simulink model "lin_kw_sim"  (R2021a)
settings: Solver=ode5  StartTime=0.0  StopTime=T  FixedStep=sim_step  RelTol=1e-3  AbsTol=1e-6
values from neighbouring files (symbols this model uses):
  f = Fk/(M*g)    [ideal_pendulum.m]    (also in lin_kw.m = 0.00027344; rms_calc.m = 1e-05)
  g = 9.81    [ideal_pendulum.m]    (also in lin_kw.m; non_lin_inv_pend_sim_real.m; non_lin_inverted_pendulum.m; non_lin_model_compare.m)
  J = 0.0038583    [lin_kw.m]
  l = g*((mean_period/(2*pi))^2)    [ideal_pendulum.m]    (also in lin_kw.m = 0.01955717; non_lin_inv_pend_sim_real.m = 1; non_lin_model_compare.m = 1e-05; rms_calc.m = 0.001)
  M = 0.5723 + 0.12    (= 0.6923)    [ideal_pendulum.m]    (also in lin_kw.m = 0.5723; non_lin_inv_pend_sim_real.m = 1; non_lin_inverted_pendulum.m = 0.5723; non_lin_model_compare.m = 0.5723)
  m = 0.12    [lin_kw.m]    (also in non_lin_inv_pend_sim_real.m = 0.5; non_lin_inverted_pendulum.m; non_lin_model_compare.m)
  step_value = 1    [ideal_pendulum.m]    (also in lin_kw.m = 10; rms_calc.m = 10)
libraries: slident x1
settings Model: ExtModeTrigDuration=18000  ExtModeTrigLevel=0.400000  Creator=jims  LastModifiedBy=Piotr
settings SolverCC: AutoScaleAbsTol=off
settings DataIOCC: ExternalInput=[]  InitialState=[]  MaxDataPoints=5000  SaveFormat=Array  SignalLoggingSaveFormat=ModelDataLogs  SaveOutput=off  SaveTime=off  ReturnWorkspaceOutputs=off
settings OptimizationCC: BooleanDataType=off  ExpressionDepthLimit=2147483647  LifeSpan=inf
settings DebuggingCC: SaveWithParameterizedLinksMsg=none  UnderspecifiedInitializationDetection=Classic  MergeDetectMultiDrivingBlocksExec=none  SignalResolutionControl=TryResolveAllWithWarning  MultiTaskDSMMsg=warning  MultiTaskCondExecSysMsg=none  IntegerOverflowMsg=none  FcnCallInpInsideContextMsg=warning  StateNameClashWarn=warning  SFUnexpectedBacktrackingDiag=warning  SFNoUnconditionalDefaultTransitionDiag=warning  SFExecutionAtInitializationDiag=none  SFMachineParentedDataDiag=warning  IntegerSaturationMsg=none  ArithmeticOperatorsInVariantConditions=warning
settings HardwareCC: TargetBitPerLong=64  TargetBitPerPointer=64  TargetIntDivRoundTo=Zero  TargetEndianess=LittleEndian  TargetWordSize=64  TargetHWDeviceType=Intel->x86-64
settings ModelReferenceCC: PropagateSignalLabelsOutOfModel=off
settings SFSimCC: SimUseLocalCustomCode=off  CustomCodeUndefinedFunction=UseInterfaceOnly
settings RTWCC: Description=Simulink Desktop Real-Time  SystemTargetFile=sldrt.tlc  TemplateMakefile=sldrt.tmf  RTWUseLocalCustomCode=off  RTWCompilerOptimization=on
settings CodeAppCC: MaxIdLength=95  StateflowObjectComments=on
settings SimulinkDesktopRealTimeCC: TargetPreCompLibLocation=C:\Program Files\MATLAB\R2021a\toolbox\sldrt\lib\win64  TargetLangStandard=C89/C90 (ANSI)  SupportVariableSizeSignals=off
settings ConfigComp: CovMetricSettings=dw  CovSaveCumulativeToWorkspaceVar=on  CovSaveSingleToWorkspaceVar=on  CovExternalEMLEnable=off  CovSFcnEnable=off

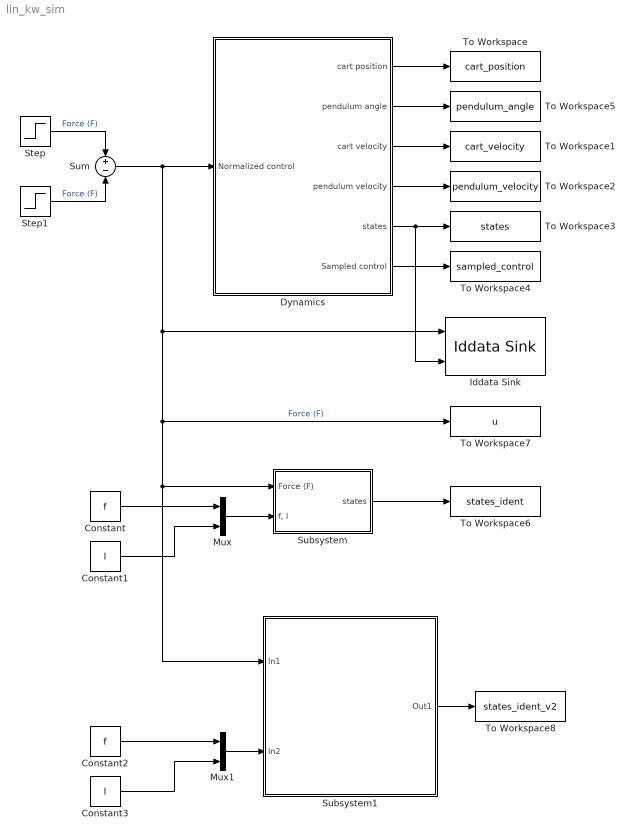
== system lin_kw_sim ==
  Constant : Constant  Value=f
  Constant1 : Constant  Value=l
  Constant2 : Constant  Value=f
  Constant3 : Constant  Value=l
  Dynamics : Subsystem  mask(Dynamics){x_ini=[0, pi, 0, 0], m=[0.5723, 0.12], fr=[0.00027344,  1.1975875,  0.5], P4=[0.01955717, 0.0038583, 9.81], Up=[ 12.86, 0.093125], DZ=[0.1, 1.5]}
      mask prompts: x_ini "Initial state vector [x1(0)  x2(0)  x3(0)  x4(0)]"; m "mass of cart (mc)  mass of pendulum (mp)"; fr "friction :  fp  FS  FC"; P4 "Distance (l), Total Inertia moment (J), gravity (g)"; Up "control : magnitude (M)    DZu"; DZ "minimal velocities : cart (DZcv)  pendulum (DZcp)"
      mask help:
      | Pendulum-Cart Dynamics
      |
      | Copyright INTECO 1997
      mask init:
      | DZcv=DZ(1);DZcp=DZ(2);DZu=Up(2);l=P4(1);J=P4(2);g=P4(3);M=Up(1);mc=m(1);mp=m(2);fp=fr(1);FS=fr(2);FC=fr(3);mi=l*(mc+mp);a=l*l+J/(mc+mp);
      mask Display: plot(0,0,100,100,[40,48,48,40,40],[60,60,49,49,60],[37,44],[9,54],[100,8,4,1,0,100,100,0,40,100,100,0,0,40],[44,44,44,44,45,46,45,44,45,45,43,43,46,46],[100,48],[55,55],[0,40],[55,55])
  Iddata Sink : slident/Iddata Sink  datasetname=data  Ts=0.1  isu=on  isy=on
      settings: SourceProductBaseCode=ID
  Mux : Mux  Inputs=2
  Mux1 : Mux  Inputs=2
  Step : Step  After=step_value  SampleTime=0
  Step1 : Step  Time=1.01  After=step_value  SampleTime=0
  Subsystem : Subsystem
  Subsystem1 : Subsystem
  Sum : Sum  Inputs=+|-
  To Workspace : ToWorkspace  VariableName=cart_position  SampleTime=-1
  To Workspace1 : ToWorkspace  VariableName=cart_velocity  SampleTime=-1
  To Workspace2 : ToWorkspace  VariableName=pendulum_velocity  SampleTime=-1
  To Workspace3 : ToWorkspace  VariableName=states  SampleTime=-1
  To Workspace4 : ToWorkspace  VariableName=sampled_control  SampleTime=-1
  To Workspace5 : ToWorkspace  VariableName=pendulum_angle  SampleTime=-1
  To Workspace6 : ToWorkspace  VariableName=states_ident  SampleTime=-1
  To Workspace7 : ToWorkspace  VariableName=u  SampleTime=-1
  To Workspace8 : ToWorkspace  VariableName=states_ident_v2  SampleTime=-1
  wires:
  Dynamics/1(cart position) -> To Workspace/1
  Dynamics/2(pendulum angle) -> To Workspace5/1
  Dynamics/6(Sampled control) -> To Workspace4/1
  Dynamics/4(pendulum velocity) -> To Workspace2/1
  Dynamics/3(cart velocity) -> To Workspace1/1
  Dynamics/5(states) -> Iddata Sink/2, To Workspace3/1
  Sum/1 -> Subsystem1/1(In1), Subsystem/1(Force (F)), To Workspace7/1, Iddata Sink/1, Dynamics/1(Normalized control)  "Force (F)"
  Subsystem/1(states) -> To Workspace6/1
  Constant/1 -> Mux/1
  Constant1/1 -> Mux/2
  Mux/1 -> Subsystem/2("f, l")
  Step1/1 -> Sum/2  "Force (F)"
  Step/1 -> Sum/1  "Force (F)"
  Constant3/1 -> Mux1/2
  Constant2/1 -> Mux1/1
  Mux1/1 -> Subsystem1/2(In2)
  Subsystem1/1(Out1) -> To Workspace8/1

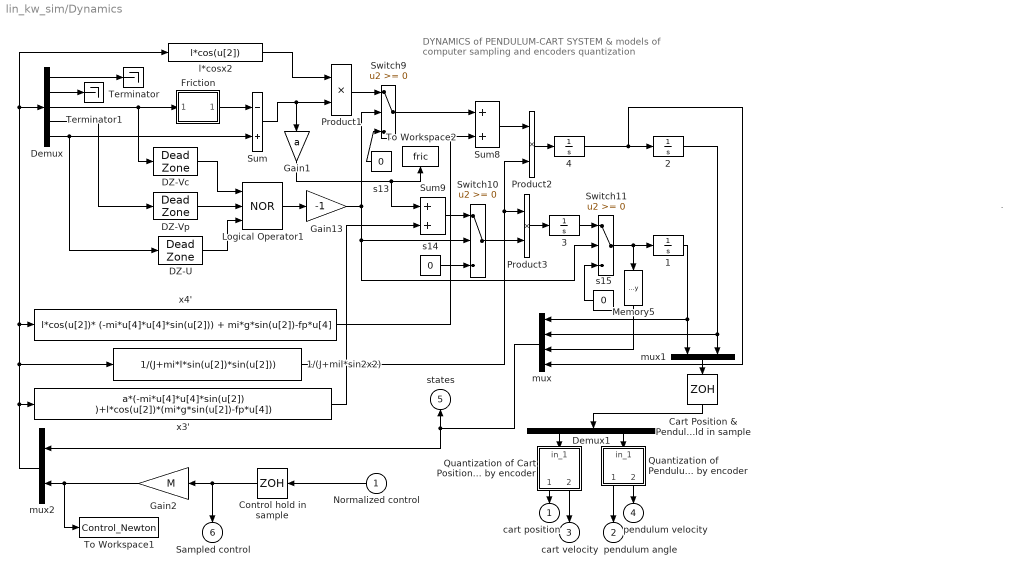
== system lin_kw_sim/Dynamics ==
  note: DYNAMICS of
      | PENDULUM-CART SYSTEM
      | & models of
      | computer sampling and encoders quantization
  note: .
  Normalized control : Inport
  " Quantization of Pendulum Angle introduced by encoder" : Subsystem
  1 : Integrator  InitialCondition=x_ini(1)
  1/(J+mil*sin2x2) : Fcn  Expr=1/(J+mi*l*sin(u[2])*sin(u[2]))
  2 : Integrator  InitialCondition=x_ini(2)
  3 : Integrator  InitialCondition=x_ini(3)
  4 : Integrator  InitialCondition=x_ini(4)
  Cart Position & Pendulum Angle hold in sample : ZeroOrderHold  SampleTime=0.01
  Control hold in sample : ZeroOrderHold  SampleTime=0.01
  DZ-U : DeadZone  LowerValue=-DZu  UpperValue=DZu  SaturateOnIntegerOverflow=on
  DZ-Vc : DeadZone  LowerValue=-DZcv  UpperValue=DZcv  SaturateOnIntegerOverflow=on
  DZ-Vp : DeadZone  LowerValue=-DZcp  UpperValue=DZcp  SaturateOnIntegerOverflow=on
  Demux : Demux  Outputs=5
      settings: DisplayOption=none
  Demux1 : Demux  Outputs=2
      settings: DisplayOption=none
  Friction : Subsystem  mask(Coulombic and Viscous Friction){FS=FS, FC=FC}
      mask prompts: FS "Static friction"; FC "Coulomb friction"
      mask help:
      | A discontinuity offset at zero models coulomb friction.  Linear gain models viscous friction.
      | y = sign(x) * (Umax * abs(x) + friction)
      mask Help:
      | This block has a discontinuity
      | at zero and a linear gain afterward.
      | y= sign(x)*(Umax*abs(x)+friction)
  Gain1 : Gain  Gain=a  SaturateOnIntegerOverflow=on  OutDataTypeStr=Inherit: Same as input  ParamDataTypeStr=Inherit: Same as input
  Gain13 : Gain  Gain=-1  SaturateOnIntegerOverflow=on  OutDataTypeStr=Inherit: Same as input  ParamDataTypeStr=Inherit: Same as input
  Gain2 : Gain  Gain=M  SaturateOnIntegerOverflow=on  OutDataTypeStr=Inherit: Same as input  ParamDataTypeStr=Inherit: Same as input
  Logical Operator1 : Logic  Operator=NOR  Inputs=3
  Memory5 : Memory
  Product1 : Product  InputSameDT=on  RndMeth=Zero  SaturateOnIntegerOverflow=on  OutDataTypeStr=Inherit: Same as first input
  Product2 : Product  InputSameDT=on  RndMeth=Zero  SaturateOnIntegerOverflow=on  OutDataTypeStr=Inherit: Same as first input
  Product3 : Product  InputSameDT=on  RndMeth=Zero  SaturateOnIntegerOverflow=on  OutDataTypeStr=Inherit: Same as first input
  "Quantization of Cart Position introduced by encoder " : Subsystem
  Sum : Sum  Inputs=-+  InputSameDT=on  SaturateOnIntegerOverflow=on  OutDataTypeStr=Inherit: Same as first input
  Sum8 : Sum  InputSameDT=on  SaturateOnIntegerOverflow=on  OutDataTypeStr=Inherit: Same as first input
  Sum9 : Sum  InputSameDT=on  SaturateOnIntegerOverflow=on  OutDataTypeStr=Inherit: Same as first input
  Switch10 : Switch  SaturateOnIntegerOverflow=on  InputSameDT=on
  Switch11 : Switch  SaturateOnIntegerOverflow=on  InputSameDT=on
  Switch9 : Switch  SaturateOnIntegerOverflow=on  InputSameDT=on
  Terminator : Terminator
  Terminator1 : Terminator
  To Workspace1 : ToWorkspace  VariableName=Control_Newton
      settings: MaxDataPoints=100000
  To Workspace2 : ToWorkspace  VariableName=fric
      settings: MaxDataPoints=100000
  l*cosx2 : Fcn  Expr=l*cos(u[2])
  mux : Mux
  mux1 : Mux  Inputs=2
  mux2 : Mux  Inputs=[4 1]
  s13 : Constant  Value=0
  s14 : Constant  Value=0
  s15 : Constant  Value=0
  x3' : Fcn  Expr=a*(-mi*u[4]*u[4]*sin(u[2]) )+l*cos(u[2])*(mi*g*sin(u[2])-fp*u[4])
  x4' : Fcn  Expr=l*cos(u[2])* (-mi*u[4]*u[4]*sin(u[2])) + mi*g*sin(u[2])-fp*u[4]
  cart position : Outport  InitialOutput=0
  pendulum angle : Outport  Port=2  InitialOutput=0
  cart velocity : Outport  Port=3  InitialOutput=0
  pendulum velocity : Outport  Port=4  InitialOutput=0
  states : Outport  Port=5  InitialOutput=0
  Sampled control : Outport  Port=6  InitialOutput=0
  wires:
  Demux1/1 -> "Quantization of Cart Position introduced by encoder "/1(in_1)
  mux/1 -> mux2/1, states/1
  "Quantization of Cart Position introduced by encoder "/1(out_1) -> cart position/1
  "Quantization of Cart Position introduced by encoder "/2(out_2) -> cart velocity/1
  " Quantization of Pendulum Angle introduced by encoder"/1(out_1) -> pendulum angle/1
  " Quantization of Pendulum Angle introduced by encoder"/2(out_2) -> pendulum velocity/1
  Demux1/2 -> " Quantization of Pendulum Angle introduced by encoder"/1(in_1)
  Control hold in sample/1 -> Sampled control/1, Gain2/1
  Normalized control/1 -> Control hold in sample/1
  Cart Position & Pendulum Angle hold in sample/1 -> Demux1/1
  mux1/1 -> Cart Position & Pendulum Angle hold in sample/1
  1/1 -> mux1/1, mux/1
  2/1 -> mux1/2, mux/2
  4/1 -> mux/4, 2/1
  Switch11/1 -> Memory5/1, 1/1
  Memory5/1 -> mux/3
  Demux/2 -> Terminator1/1
  Demux/5 -> DZ-U/1, Sum/2
  Demux/1 -> Terminator/1
  Demux/4 -> DZ-Vp/1
  Demux/3 -> DZ-Vc/1, Friction/1(In1)
  DZ-U/1 -> Logical Operator1/3
  Logical Operator1/1 -> Gain13/1
  DZ-Vp/1 -> Logical Operator1/2
  DZ-Vc/1 -> Logical Operator1/1
  l*cosx2/1 -> Product1/1
  s13/1 -> Switch9/3
  Switch9/1 -> Sum8/1
  s14/1 -> Switch10/3
  Product1/1 -> Switch9/1
  x4'/1 -> Sum8/2
  Sum8/1 -> Product2/1
  Product2/1 -> 4/1
  Product3/1 -> 3/1
  Sum9/1 -> Switch10/1
  3/1 -> Switch11/1
  s15/1 -> Switch11/3
  Gain13/1 -> Switch9/2, Switch11/2, Switch10/2
  Switch10/1 -> Product3/2
  Sum/1 -> Product1/2, Gain1/1
  mux2/1 -> x3'/1, Demux/1, l*cosx2/1, x4'/1, 1/(J+mil*sin2x2)/1
  x3'/1 -> Sum9/2
  1/(J+mil*sin2x2)/1 -> Product2/2, Product3/1
  Gain1/1 -> Sum9/1, To Workspace2/1
  Gain2/1 -> To Workspace1/1, mux2/2
  Friction/1(Out1) -> Sum/1

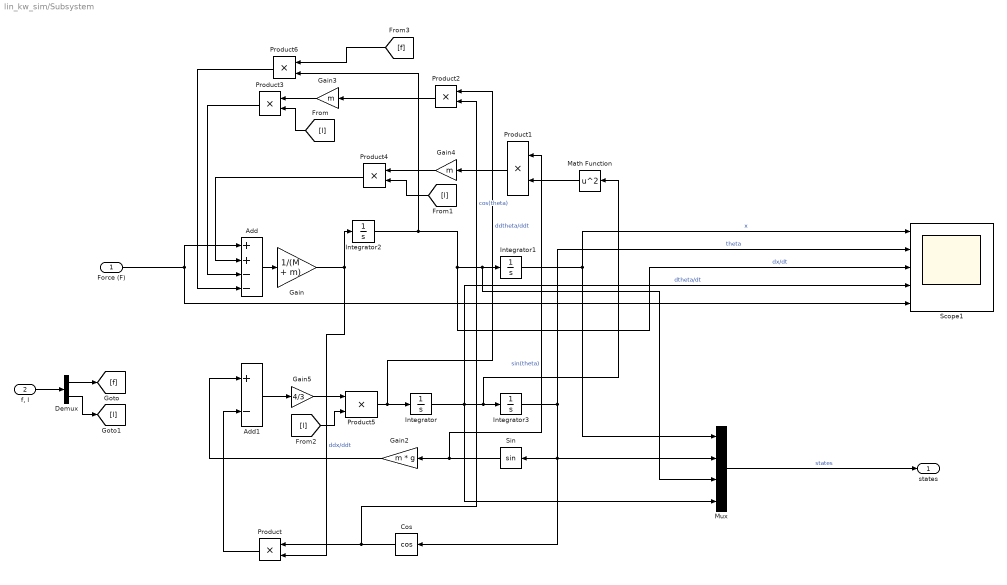
== system lin_kw_sim/Subsystem ==
  Force (F) : Inport
  "f, l" : Inport  Port=2
  Add : Sum  Inputs=++--
  Add1 : Sum  Inputs=+-
  Cos : Trigonometry  Operator=cos
  Demux : Demux  Outputs=2
  Gain : Gain  Gain=1/(M + m)
  Gain2 : Gain  Gain=m * g
  Gain3 : Gain  Gain=m
  Gain4 : Gain  Gain=m
  Gain5 : Gain  Gain=4/3
  Integrator : Integrator
  Integrator1 : Integrator
  Integrator2 : Integrator
  Integrator3 : Integrator  InitialCondition=pi
  Math Function : Math  Operator=square  SaturateOnIntegerOverflow=on
  Mux : Mux
  Product{,1..6} (7 alike) : Product
  Scope1 : Scope  NumInputPorts=5
  Sin : Trigonometry
  states : Outport
  wires:
  Product/1 -> Add1/2
  Integrator3/1 -> Scope1/2, Cos/1, Sin/1, Mux/2  "theta"
  Integrator/1 -> Scope1/4, Math Function/1, Integrator3/1, Mux/4  "dtheta/dt"
  Integrator1/1 -> Mux/1, Scope1/1  "x"
  Cos/1 -> Product2/2, Product/1  "cos(theta)"
  Gain/1 -> Product/2, Integrator2/1  "ddx/ddt"
  Add/1 -> Gain/1
  Add1/1 -> Gain5/1
  Integrator2/1 -> Mux/3, Integrator1/1, Scope1/3, Product6/2  "dx/dt"
  Math Function/1 -> Product1/2
  Sin/1 -> Gain2/1, Product1/1  "sin(theta)"
  Force (F)/1 -> Add/1, Scope1/5
  Mux/1 -> states/1  "states"
  Product6/1 -> Add/4
  Gain2/1 -> Add1/1
  Product5/1 -> Product2/1, Integrator/1  "ddtheta/ddt"
  Product4/1 -> Add/2
  Product3/1 -> Add/3
  Product1/1 -> Gain4/1
  "f, l"/1 -> Demux/1
  Demux/1 -> [f]
  Demux/2 -> [l]
  Gain3/1 -> Product3/1
  Product2/1 -> Gain3/1
  [l] -> Product3/2
  Gain4/1 -> Product4/1
  [l] -> Product4/2
  Gain5/1 -> Product5/1
  [l] -> Product5/2
  [f] -> Product6/1

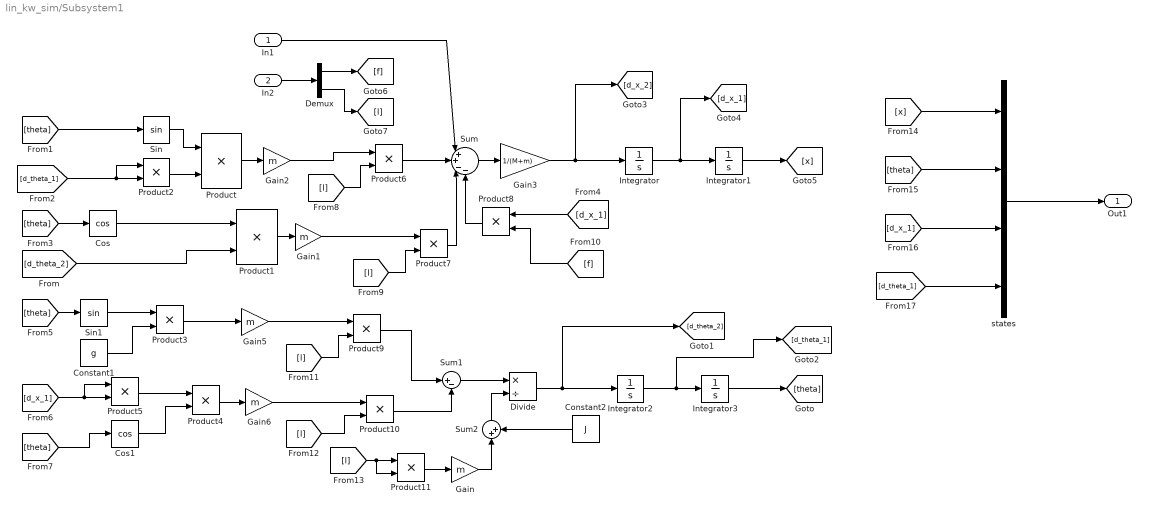
== system lin_kw_sim/Subsystem1 ==
  In1 : Inport
  In2 : Inport  Port=2
  Constant1 : Constant  Value=g
  Constant2 : Constant  Value=J
  Cos : Trigonometry  Operator=cos
  Cos1 : Trigonometry  Operator=cos
  Demux : Demux  Outputs=2
  Divide : Product  Inputs=*/
  Gain{,1..2,5..6} (5 alike) : Gain  Gain=m
  Gain3 : Gain  Gain=1/(M+m)
  Integrator : Integrator
  Integrator1 : Integrator
  Integrator2 : Integrator
  Integrator3 : Integrator  InitialCondition=pi
  Product{,1..11} (12 alike) : Product
  Sin : Trigonometry
  Sin1 : Trigonometry
  Sum : Sum  Inputs=|++--
  Sum1 : Sum  Inputs=|+-
  Sum2 : Sum  Inputs=|++
  states : Mux
  Out1 : Outport
  wires:
  Sum/1 -> Gain3/1
  [theta] -> Cos1/1
  In1/1 -> Sum/1
  Sum1/1 -> Divide/1
  Integrator2/1 -> [d_theta_1], Integrator3/1
  Integrator/1 -> [d_x_1], Integrator1/1
  Product5/1 -> Product4/1
  [d_x_1] -> Product5/1, Product5/2
  [theta] -> Sin1/1
  Cos1/1 -> Product4/2
  Constant1/1 -> Product3/2
  Sin1/1 -> Product3/1
  Product2/1 -> Product/2
  [theta] -> Cos/1
  Gain3/1 -> [d_x_2], Integrator/1
  Product/1 -> Gain2/1
  [d_theta_1] -> Product2/1, Product2/2
  [d_theta_2] -> Product1/2
  Cos/1 -> Product1/1
  Product8/1 -> Sum/4
  Integrator1/1 -> [x]
  Integrator3/1 -> [theta]
  [d_x_1] -> Product8/1
  Product1/1 -> Gain1/1
  Divide/1 -> Integrator2/1, [d_theta_2]
  Sin/1 -> Product/1
  [theta] -> Sin/1
  Demux/2 -> [l]
  In2/1 -> Demux/1
  Demux/1 -> [f]
  Gain2/1 -> Product6/1
  Product6/1 -> Sum/2
  [l] -> Product6/2
  Gain1/1 -> Product7/1
  [l] -> Product7/2
  Product7/1 -> Sum/3
  [f] -> Product8/2
  Gain5/1 -> Product9/1
  [l] -> Product9/2
  Product3/1 -> Gain5/1
  Product9/1 -> Sum1/1
  Gain6/1 -> Product10/1
  [l] -> Product10/2
  Product4/1 -> Gain6/1
  Product10/1 -> Sum1/2
  Sum2/1 -> Divide/2
  [l] -> Product11/2, Product11/1
  Product11/1 -> Gain/1
  Gain/1 -> Sum2/1
  Constant2/1 -> Sum2/2
  [x] -> states/1
  [theta] -> states/2
  [d_x_1] -> states/3
  [d_theta_1] -> states/4
  states/1 -> Out1/1

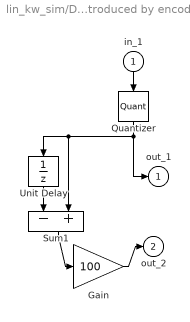
== system lin_kw_sim/Dynamics/ Quantization of Pendulum Angle introduced by encoder ==
  in_1 : Inport
  Gain : Gain  Gain=100  SaturateOnIntegerOverflow=on  OutDataTypeStr=Inherit: Same as input  ParamDataTypeStr=Inherit: Same as input
  Quantizer : Quantizer  QuantizationInterval=0.001534
  Sum1 : Sum  Inputs=-+  InputSameDT=on  SaturateOnIntegerOverflow=on  OutDataTypeStr=Inherit: Same as first input
  Unit Delay : UnitDelay  InitialCondition=x_ini(2)  SampleTime=0.01  HasFrameUpgradeWarning=on
  out_1 : Outport  InitialOutput=0
  out_2 : Outport  Port=2  InitialOutput=0
  wires:
  in_1/1 -> Quantizer/1
  Quantizer/1 -> Sum1/2, Unit Delay/1, out_1/1
  Sum1/1 -> Gain/1
  Gain/1 -> out_2/1
  Unit Delay/1 -> Sum1/1

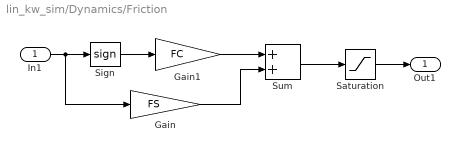
== system lin_kw_sim/Dynamics/Friction ==
  In1 : Inport
  Gain : Gain  Gain=FS  SaturateOnIntegerOverflow=on  OutDataTypeStr=Inherit: Same as input  ParamDataTypeStr=Inherit: Same as input
  Gain1 : Gain  Gain=FC  SaturateOnIntegerOverflow=on  OutDataTypeStr=Inherit: Same as input  ParamDataTypeStr=Inherit: Same as input
  Saturation : Saturate  UpperLimit=1  LowerLimit=-1
  Sign : Signum
  Sum : Sum  InputSameDT=on  SaturateOnIntegerOverflow=on  OutDataTypeStr=Inherit: Same as first input
  Out1 : Outport  InitialOutput=0
  wires:
  Saturation/1 -> Out1/1
  Sum/1 -> Saturation/1
  Sign/1 -> Gain1/1
  In1/1 -> Gain/1, Sign/1
  Gain1/1 -> Sum/1
  Gain/1 -> Sum/2

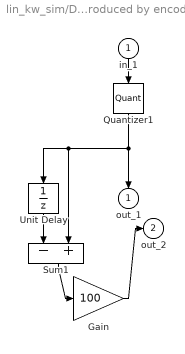
== system lin_kw_sim/Dynamics/Quantization of Cart Position introduced by encoder  ==
  in_1 : Inport
  Gain : Gain  Gain=100  SaturateOnIntegerOverflow=on  OutDataTypeStr=Inherit: Same as input  ParamDataTypeStr=Inherit: Same as input
  Quantizer1 : Quantizer  QuantizationInterval=5.7053e-005
  Sum1 : Sum  Inputs=-+  InputSameDT=on  SaturateOnIntegerOverflow=on  OutDataTypeStr=Inherit: Same as first input
  Unit Delay : UnitDelay  InitialCondition=x_ini(1)  SampleTime=0.01  HasFrameUpgradeWarning=on
  out_1 : Outport  InitialOutput=0
  out_2 : Outport  Port=2  InitialOutput=0
  wires:
  Quantizer1/1 -> Sum1/2, Unit Delay/1, out_1/1
  Unit Delay/1 -> Sum1/1
  Gain/1 -> out_2/1
  in_1/1 -> Quantizer1/1
  Sum1/1 -> Gain/1
